simulink model "plant"  (R2022b)
settings: Solver=VariableStepAuto  StartTime=0.0  StopTime=100  RelTol=1e-3
values from neighbouring files (symbols this model uses):
  veh_params = get_vehicle_params    [init_plant.m]
undefined symbols (not defined in the file or in its folder): accel_body_mps2, body_ang_acc_radps2, body_rates_radps, dcm_ned_2_body, euler_ang_rad, pos_ned_m, v_body_mps, v_ned_mps
libraries: shared6dof x1, main_rotor x1
settings Model: DataDictionary=plant_data.sldd  Creator=Tanmay.Mandal  LastModifiedBy=Tanmay.Mandal

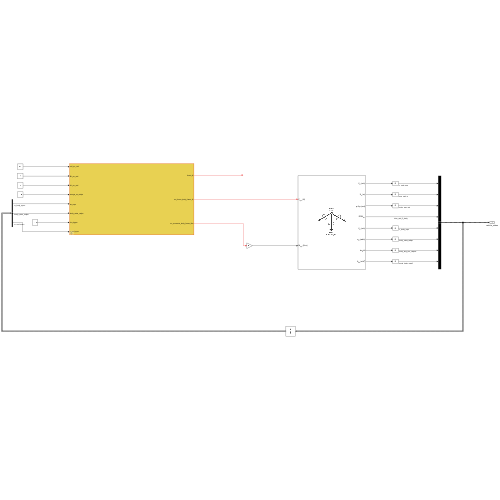
[thumbnail: Simulink's stored preview of the top-level diagram]
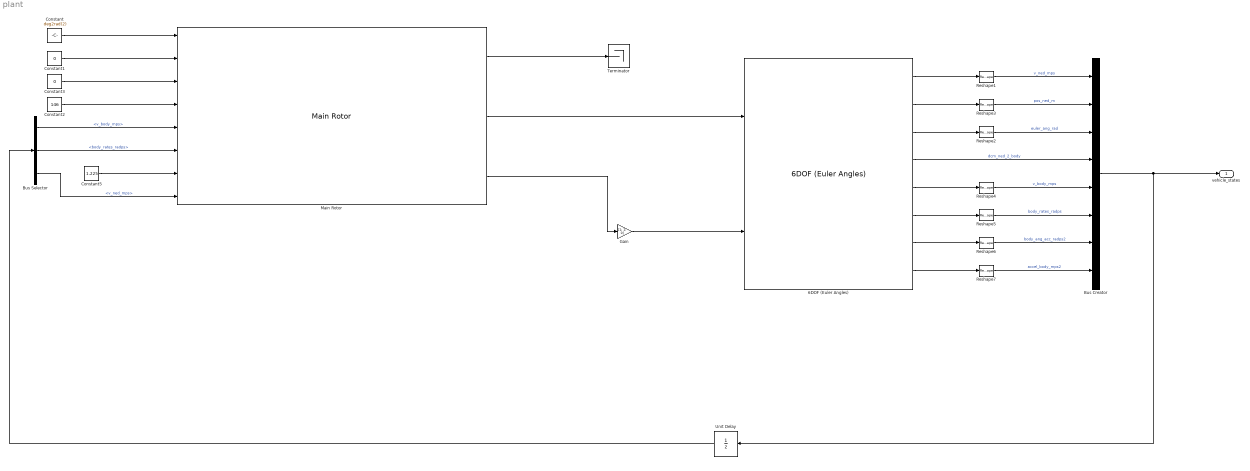
== system plant ==
  6DOF (Euler Angles) : shared6dof/6DOF (Euler Angles)  units=Metric (MKS)  mtype=Fixed  rep=Euler Angles  xme_0=[0 0 0]  Vm_0=[0 0 0]  eul_0=[0 0 0]  pm_0=[0 0 0]  mass_0=veh_params.mass_kg  mass_e=0.5  mass_f=2.0  inertia=veh_params.inertia_kgm2*100  inertia_e=eye(3)  inertia_f=2*eye(3)  k_quat=1.0  vre_flag=on  abi_flag=off  aMode=0  xme_statename=''  Vm_statename=''  eul_statename=''  quat_statename=''  pm_statename=''  mass_statename=''
  Bus Creator : BusCreator  Inputs=v_ned_mps,pos_ned_m,euler_ang_rad,dcm_ned_2_body,v_body_mps,body_rates_radps,body_ang_acc_radps2,accel_body_mps2  OutDataTypeStr=Bus: vehicle_state_bus  NonVirtualBus=on
  Bus Selector : BusSelector  OutputSignals=v_body_mps,body_rates_radps,v_ned_mps
  Constant : Constant  Value=deg2rad(2)
  Constant1 : Constant  Value=0
  Constant2 : Constant  Value=146
  Constant3 : Constant  Value=0
  Constant5 : Constant  Value=1.225
  Gain : Gain  Gain=[1; 1; 0]
  Main Rotor : main_rotor/Main Rotor  veh_params=veh_params  universal_constants=universal_constants
  Reshape{1..7} (7 alike) : Reshape  OutputDimensionality=Customize  OutputDimensions=[3, 1]
  Terminator : Terminator
  Unit Delay : UnitDelay  SampleTime=-1  HasFrameUpgradeWarning=on
  vehicle_states : Outport  OutDataTypeStr=Bus: vehicle_state_bus  BusOutputAsStruct=on
  wires:
  Main Rotor/1 -> Terminator/1
  Main Rotor/2 -> 6DOF (Euler Angles)/1
  Main Rotor/3 -> Gain/1
  Constant/1 -> Main Rotor/1
  Constant1/1 -> Main Rotor/2
  Constant2/1 -> Main Rotor/4
  Bus Selector/1 -> Main Rotor/5  "<v_body_mps>"
  Bus Selector/2 -> Main Rotor/6  "<body_rates_radps>"
  Constant5/1 -> Main Rotor/7
  Bus Selector/3 -> Main Rotor/8  "<v_ned_mps>"
  6DOF (Euler Angles)/1 -> Reshape1/1
  6DOF (Euler Angles)/2 -> Reshape3/1
  6DOF (Euler Angles)/3 -> Reshape2/1
  6DOF (Euler Angles)/4 -> Bus Creator/4  "dcm_ned_2_body"
  6DOF (Euler Angles)/5 -> Reshape4/1
  6DOF (Euler Angles)/6 -> Reshape5/1
  6DOF (Euler Angles)/7 -> Reshape6/1
  6DOF (Euler Angles)/8 -> Reshape7/1
  Bus Creator/1 -> Unit Delay/1, vehicle_states/1
  Reshape1/1 -> Bus Creator/1  "v_ned_mps"
  Reshape2/1 -> Bus Creator/3  "euler_ang_rad"
  Reshape3/1 -> Bus Creator/2  "pos_ned_m"
  Reshape4/1 -> Bus Creator/5  "v_body_mps"
  Reshape5/1 -> Bus Creator/6  "body_rates_radps"
  Reshape6/1 -> Bus Creator/7  "body_ang_acc_radps2"
  Reshape7/1 -> Bus Creator/8  "accel_body_mps2"
  Unit Delay/1 -> Bus Selector/1
  Gain/1 -> 6DOF (Euler Angles)/2
  Constant3/1 -> Main Rotor/3
